simulink model "LotkaVolterraCap"  (R2020a)
settings: Solver=ode45  StartTime=0.0  StopTime=Time  RelTol=1e-3
undefined symbols (not defined in the file): beta, D0, delta, gamma, k, P0, r
settings Model: Creator=mluser  LastModifiedBy=curie
settings DataIOCC: ReturnWorkspaceOutputs=off

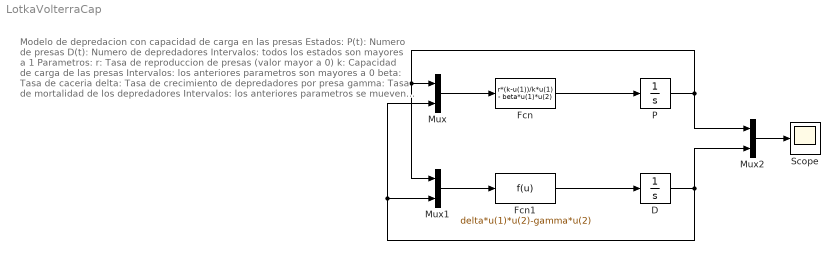
== system LotkaVolterraCap ==
  note: Modelo de depredacion con capacidad de carga en
      | las presas
      |
      | Estados:
      | P(t): Numero de presas
      | D(t): Numero de depredadores
      |
      | Intervalos: todos los estados son mayores a 1
      |
      | Parametros:
      | r: Tasa de reproduccion de presas (valor mayor a 0)
      | k: Capacidad de carga de las presas
      |
      | Intervalos: los anteriores parametros son mayores a 0
      |
      | beta: Tasa de caceria
      | delta: Tasa de crecimiento de depredadores por presa
      | gamma: Tasa de mortalidad de los depredadores
      |
      | Intervalos: los anteriores parametros se
      | mueven entre 0 y1
  D : Integrator  InitialCondition=D0
  Fcn : Fcn  Expr=r*(k-u(1))/k*u(1) - beta*u(1)*u(2)
  Fcn1 : Fcn  Expr=delta*u(1)*u(2)-gamma*u(2)
  Mux : Mux  Inputs=2
  Mux1 : Mux  Inputs=2
  Mux2 : Mux  Inputs=2
  P : Integrator  InitialCondition=P0
  Scope : Scope
  wires:
  Mux2/1 -> Scope/1
  Fcn1/1 -> D/1
  P/1 -> Mux1/1, Mux/1, Mux2/1
  D/1 -> Mux1/2, Mux/2, Mux2/2
  Fcn/1 -> P/1
  Mux1/1 -> Fcn1/1
  Mux/1 -> Fcn/1
